simulink model "EnabledSubsystem_modelC"  (R2018b)
settings: Solver=FixedStepAuto  StartTime=0.0  StopTime=tFinal  FixedStep=deltaT  RelTol=1e-3
values from neighbouring files (symbols this model uses):
  V_rel_b = [0;0;0]    [MAIN_EnabledSubsystem.m]
libraries: UWAerospaceBlockset_Utilities x1
settings Model: Creator=Christopher  LastModifiedBy=Christopher

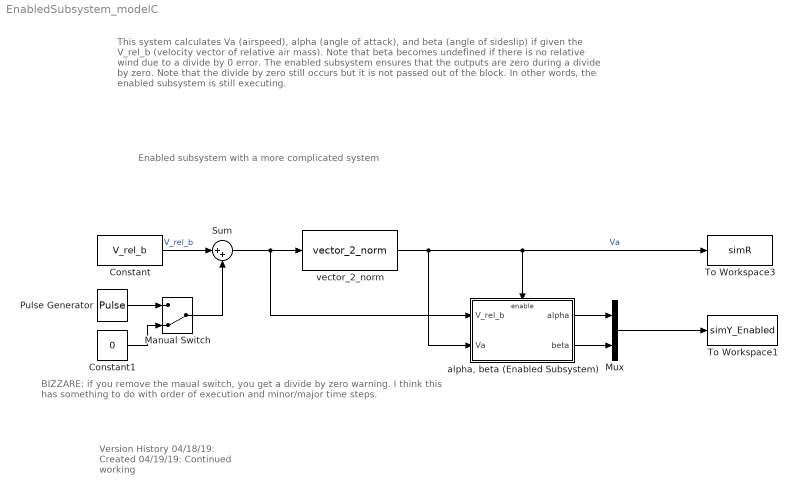
== system EnabledSubsystem_modelC ==
  note: BIZZARE: if you remove the maual switch, you get a divide by zero warning.
      | I think this has something to do with order of execution and minor/major time steps.
  note: Enabled subsystem with a more complicated system
  note: This system calculates Va (airspeed), alpha (angle of attack), and beta (angle of sideslip) if given the V_rel_b (velocity vector of relative air mass).
      |
      | Note that beta becomes undefined if there is no relative wind due to a divide by 0 error.
      |
      | The enabled subsystem ensures that the outputs are zero during a divide by zero.  Note that the divide by zero still occurs but it is not passed out of the block.  In other words, the enabled subsystem is still executing.
  note: Version History
      | 04/18/19: Created
      | 04/19/19: Continued working
  Constant : Constant  Value=V_rel_b
  Constant1 : Constant  Value=0
  Manual Switch : ManualSwitch  CurrentSetting=0
  Mux : Mux  Inputs=2
  Pulse Generator : DiscretePulseGenerator  PulseType=Time based  Period=.5  PulseWidth=70
  Sum : Sum  Inputs=|++
  To Workspace1 : ToWorkspace  VariableName=simY_Enabled  SaveFormat=Timeseries  SampleTime=-1
  To Workspace3 : ToWorkspace  VariableName=simR  SaveFormat=Timeseries  SampleTime=-1
  "alpha, beta (Enabled Subsystem)" : Subsystem
  vector_2_norm : UWAerospaceBlockset_Utilities/vector_2_norm
  wires:
  Mux/1 -> To Workspace1/1
  vector_2_norm/1 -> "alpha, beta (Enabled Subsystem)"/2(Va), "alpha, beta (Enabled Subsystem)"/Enable, To Workspace3/1  "Va"
  "alpha, beta (Enabled Subsystem)"/1(alpha) -> Mux/1
  "alpha, beta (Enabled Subsystem)"/2(beta) -> Mux/2
  Sum/1 -> "alpha, beta (Enabled Subsystem)"/1(V_rel_b), vector_2_norm/1
  Constant/1 -> Sum/1  "V_rel_b"
  Pulse Generator/1 -> Manual Switch/1
  Manual Switch/1 -> Sum/2
  Constant1/1 -> Manual Switch/2

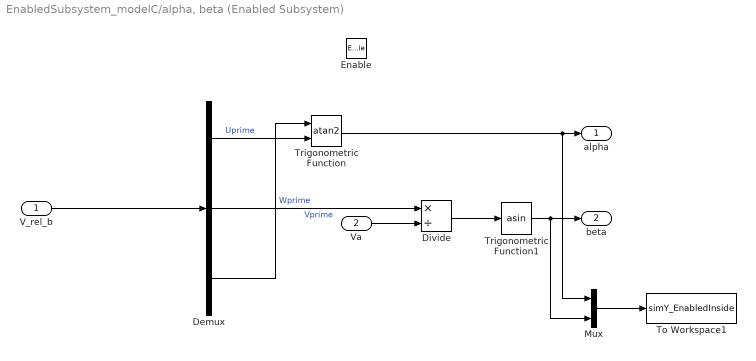
== system EnabledSubsystem_modelC/alpha, beta (Enabled Subsystem) ==
  V_rel_b : Inport
  Va : Inport  Port=2
  Enable : EnablePort
  Demux : Demux  Outputs=3
  Divide : Product  Inputs=*/
  Mux : Mux  Inputs=2
  To Workspace1 : ToWorkspace  VariableName=simY_EnabledInside  SaveFormat=Timeseries  SampleTime=-1
  Trigonometric Function : Trigonometry  Operator=atan2
  Trigonometric Function1 : Trigonometry  Operator=asin
  alpha : Outport
  beta : Outport  Port=2
  wires:
  Trigonometric Function1/1 -> Mux/2, beta/1
  V_rel_b/1 -> Demux/1
  Trigonometric Function/1 -> Mux/1, alpha/1
  Va/1 -> Divide/2
  Divide/1 -> Trigonometric Function1/1
  Demux/3 -> Trigonometric Function/1  "Wprime"
  Demux/1 -> Trigonometric Function/2  "Uprime"
  Demux/2 -> Divide/1  "Vprime"
  Mux/1 -> To Workspace1/1
